simulink model "Model_ThreePhase_SixArm"  (R2022a)
settings: Solver=VariableStepAuto  StartTime=0.0  StopTime=10.0  RelTol=1e-3
libraries: fl_lib x45
settings Model: Creator=chack  LastModifiedBy=chack

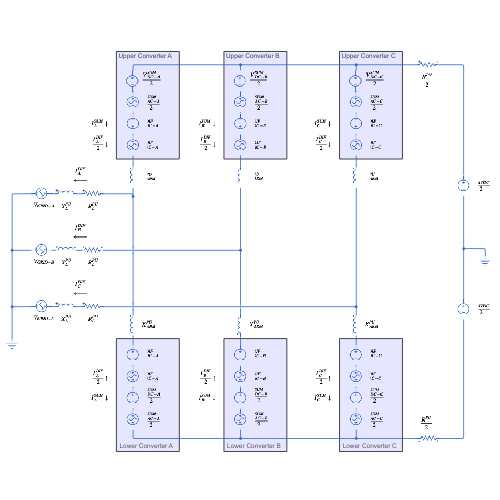
[thumbnail: Simulink's stored preview of the top-level diagram]
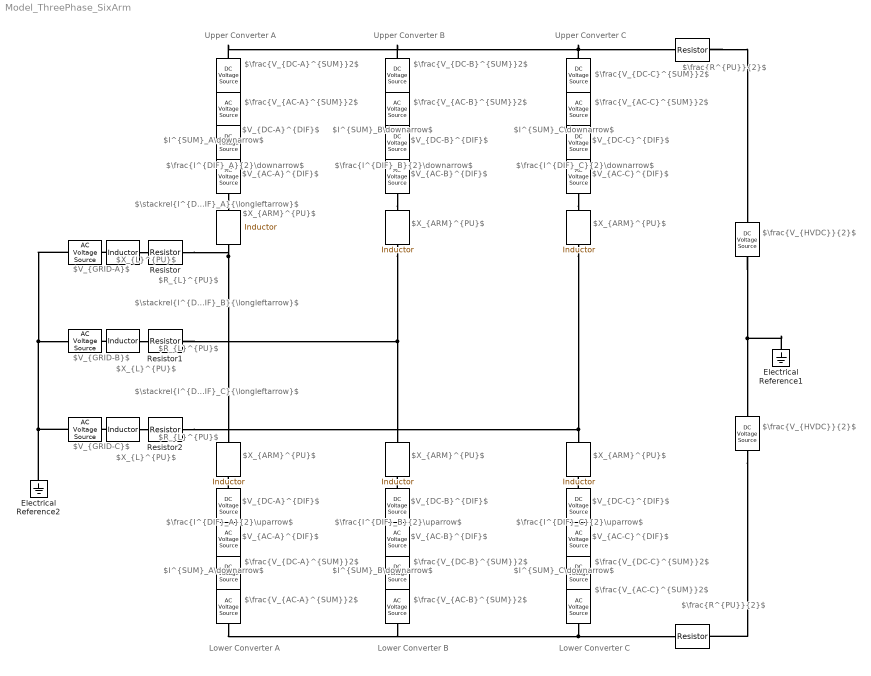
== system Model_ThreePhase_SixArm ==
  note: $I^{SUM}_A\downarrow$
  note: $\frac{I^{DIF}_A}{2}\downarrow$
  note: Lower Converter A
  note: Upper Converter A
  note: $V_{DC-A}^{DIF}$
  note: $\frac{V_{DC-A}^{SUM}}2$
  note: $V_{GRID-A}$
  note: $R_{L}^{PU}$
  note: $X_{L}^{PU}$
  note: $\frac{V_{HVDC}}{2}$
  note: $\frac{V_{HVDC}}{2}$
  note: $\frac{R^{PU}}{2}$
  note: $\frac{V_{AC-A}^{SUM}}2$
  note: $V_{AC-A}^{DIF}$
  note: $X_{ARM}^{PU}$
  note: $\frac{V_{DC-A}^{SUM}}2$
  note: $V_{DC-A}^{DIF}$
  note: $V_{AC-A}^{DIF}$
  note: $\frac{V_{AC-A}^{SUM}}2$
  note: $X_{ARM}^{PU}$
  note: $\frac{R^{PU}}{2}$
  note: $\stackrel{I^{DIF}_A}{\longleftarrow}$
  note: $\frac{I^{DIF}_A}{2}\uparrow$
  note: $I^{SUM}_A\downarrow$
  note: $X_{L}^{PU}$
  note: $V_{DC-B}^{DIF}$
  note: Lower Converter B
  note: $\frac{V_{AC-B}^{SUM}}2$
  note: $V_{AC-B}^{DIF}$
  note: $V_{DC-B}^{DIF}$
  note: $R_{L}^{PU}$
  note: $\frac{V_{AC-B}^{SUM}}2$
  note: $\frac{I^{DIF}_B}{2}\downarrow$
  note: $X_{ARM}^{PU}$
  note: $V_{AC-B}^{DIF}$
  note: $I^{SUM}_B\downarrow$
  note: $\frac{V_{DC-B}^{SUM}}2$
  note: $\frac{I^{DIF}_B}{2}\uparrow$
  note: Upper Converter B
  note: $\frac{V_{DC-B}^{SUM}}2$
  note: $X_{ARM}^{PU}$
  note: $\stackrel{I^{DIF}_B}{\longleftarrow}$
  note: $I^{SUM}_B\downarrow$
  note: $V_{GRID-B}$
  note: $X_{L}^{PU}$
  note: $V_{DC-C}^{DIF}$
  note: Lower Converter C
  note: $\frac{V_{AC-C}^{SUM}}2$
  note: $V_{AC-C}^{DIF}$
  note: $V_{DC-C}^{DIF}$
  note: $R_{L}^{PU}$
  note: $\frac{V_{AC-C}^{SUM}}2$
  note: $\frac{I^{DIF}_C}{2}\downarrow$
  note: $X_{ARM}^{PU}$
  note: $V_{AC-C}^{DIF}$
  note: $I^{SUM}_C\downarrow$
  note: $\frac{V_{DC-C}^{SUM}}2$
  note: $\frac{I^{DIF}_C}{2}\uparrow$
  note: Upper Converter C
  note: $\frac{V_{DC-C}^{SUM}}2$
  note: $X_{ARM}^{PU}$
  note: $\stackrel{I^{DIF}_C}{\longleftarrow}$
  note: $I^{SUM}_C\downarrow$
  note: $V_{GRID-C}$
  " " : fl_lib/Electrical/Electrical Sources/AC Voltage Source  amp=1 V  shift=0 deg  frequency=60 Hz  omega=0 rad/s
      settings: SourceProductBaseCode=PW,SS,VE
  "  " : fl_lib/Electrical/Electrical Elements/Inductor  l=1e-6 H  r=0 Ohm  g=1e-9 1/Ohm  i_specify=off  i_priority=None  i=0 A  i_nominal_specify=off  i_nominal_unit=A  i_nominal_value=1  v_specify=off  v_priority=None  v=0 V  v_nominal_specify=off  v_nominal_unit=V  v_nominal_value=1  i_L_specify=off  i_L_priority=High  i_L=0 A  i_L_nominal_specify=off  i_L_nominal_unit=A  i_L_nominal_value=1
      settings: SourceProductBaseCode=PW,SS,VE
  "   " : fl_lib/Electrical/Electrical Elements/Inductor  l=1e-6 H  r=0 Ohm  g=1e-9 1/Ohm  i_specify=off  i_priority=None  i=0 A  i_nominal_specify=off  i_nominal_unit=A  i_nominal_value=1  v_specify=off  v_priority=None  v=0 V  v_nominal_specify=off  v_nominal_unit=V  v_nominal_value=1  i_L_specify=off  i_L_priority=High  i_L=0 A  i_L_nominal_specify=off  i_L_nominal_unit=A  i_L_nominal_value=1
      settings: SourceProductBaseCode=PW,SS,VE
  "    " : fl_lib/Electrical/Electrical Sources/DC Voltage Source  v0=1 V
      settings: SourceProductBaseCode=PW,SS,VE
  "     " : fl_lib/Electrical/Electrical Sources/DC Voltage Source  v0=1 V
      settings: SourceProductBaseCode=PW,SS,VE
  "       " : fl_lib/Electrical/Electrical Elements/Resistor  R=1 Ohm  i_specify=off  i_priority=None  i=0 A  i_nominal_specify=off  i_nominal_unit=A  i_nominal_value=1  v_specify=off  v_priority=None  v=0 V  v_nominal_specify=off  v_nominal_unit=V  v_nominal_value=1
      settings: SourceProductBaseCode=PW,SS,VE
  "         " : fl_lib/Electrical/Electrical Elements/Resistor  R=1 Ohm  i_specify=off  i_priority=None  i=0 A  i_nominal_specify=off  i_nominal_unit=A  i_nominal_value=1  v_specify=off  v_priority=None  v=0 V  v_nominal_specify=off  v_nominal_unit=V  v_nominal_value=1
      settings: SourceProductBaseCode=PW,SS,VE
  "            " : fl_lib/Electrical/Electrical Sources/AC Voltage Source  amp=1 V  shift=0 deg  frequency=60 Hz  omega=0 rad/s
      settings: SourceProductBaseCode=PW,SS,VE
  "             " : fl_lib/Electrical/Electrical Sources/DC Voltage Source  v0=1 V
      settings: SourceProductBaseCode=PW,SS,VE
  "                " : fl_lib/Electrical/Electrical Sources/DC Voltage Source  v0=1 V
      settings: SourceProductBaseCode=PW,SS,VE
  "                 " : fl_lib/Electrical/Electrical Sources/AC Voltage Source  amp=1 V  shift=0 deg  frequency=60 Hz  omega=0 rad/s
      settings: SourceProductBaseCode=PW,SS,VE
  "                  " : fl_lib/Electrical/Electrical Sources/AC Voltage Source  amp=1 V  shift=0 deg  frequency=60 Hz  omega=0 rad/s
      settings: SourceProductBaseCode=PW,SS,VE
  "                   " : fl_lib/Electrical/Electrical Sources/AC Voltage Source  amp=1 V  shift=0 deg  frequency=60 Hz  omega=0 rad/s
      settings: SourceProductBaseCode=PW,SS,VE
  "                      " : fl_lib/Electrical/Electrical Elements/Inductor  l=1e-6 H  r=0 Ohm  g=1e-9 1/Ohm  i_specify=off  i_priority=None  i=0 A  i_nominal_specify=off  i_nominal_unit=A  i_nominal_value=1  v_specify=off  v_priority=None  v=0 V  v_nominal_specify=off  v_nominal_unit=V  v_nominal_value=1  i_L_specify=off  i_L_priority=High  i_L=0 A  i_L_nominal_specify=off  i_L_nominal_unit=A  i_L_nominal_value=1
      settings: SourceProductBaseCode=PW,SS,VE
  "                         " : fl_lib/Electrical/Electrical Sources/DC Voltage Source  v0=1 V
      settings: SourceProductBaseCode=PW,SS,VE
  "                             " : fl_lib/Electrical/Electrical Sources/DC Voltage Source  v0=1 V
      settings: SourceProductBaseCode=PW,SS,VE
  "                              " : fl_lib/Electrical/Electrical Sources/AC Voltage Source  amp=1 V  shift=0 deg  frequency=60 Hz  omega=0 rad/s
      settings: SourceProductBaseCode=PW,SS,VE
  "                                 " : fl_lib/Electrical/Electrical Sources/AC Voltage Source  amp=1 V  shift=0 deg  frequency=60 Hz  omega=0 rad/s
      settings: SourceProductBaseCode=PW,SS,VE
  "                                   " : fl_lib/Electrical/Electrical Elements/Inductor  l=1e-6 H  r=0 Ohm  g=1e-9 1/Ohm  i_specify=off  i_priority=None  i=0 A  i_nominal_specify=off  i_nominal_unit=A  i_nominal_value=1  v_specify=off  v_priority=None  v=0 V  v_nominal_specify=off  v_nominal_unit=V  v_nominal_value=1  i_L_specify=off  i_L_priority=High  i_L=0 A  i_L_nominal_specify=off  i_L_nominal_unit=A  i_L_nominal_value=1
      settings: SourceProductBaseCode=PW,SS,VE
  "                                    " : fl_lib/Electrical/Electrical Sources/DC Voltage Source  v0=1 V
      settings: SourceProductBaseCode=PW,SS,VE
  "                                     " : fl_lib/Electrical/Electrical Sources/AC Voltage Source  amp=1 V  shift=0 deg  frequency=60 Hz  omega=0 rad/s
      settings: SourceProductBaseCode=PW,SS,VE
  "                                        " : fl_lib/Electrical/Electrical Sources/DC Voltage Source  v0=1 V
      settings: SourceProductBaseCode=PW,SS,VE
  "                                         " : fl_lib/Electrical/Electrical Sources/AC Voltage Source  amp=1 V  shift=0 deg  frequency=60 Hz  omega=0 rad/s
      settings: SourceProductBaseCode=PW,SS,VE
  "                                           " : fl_lib/Electrical/Electrical Sources/AC Voltage Source  amp=1 V  shift=0 deg  frequency=60 Hz  omega=0 rad/s
      settings: SourceProductBaseCode=PW,SS,VE
  "                                              " : fl_lib/Electrical/Electrical Sources/DC Voltage Source  v0=1 V
      settings: SourceProductBaseCode=PW,SS,VE
  "                                                " : fl_lib/Electrical/Electrical Sources/AC Voltage Source  amp=1 V  shift=0 deg  frequency=60 Hz  omega=0 rad/s
      settings: SourceProductBaseCode=PW,SS,VE
  "                                                    " : fl_lib/Electrical/Electrical Elements/Inductor  l=1e-6 H  r=0 Ohm  g=1e-9 1/Ohm  i_specify=off  i_priority=None  i=0 A  i_nominal_specify=off  i_nominal_unit=A  i_nominal_value=1  v_specify=off  v_priority=None  v=0 V  v_nominal_specify=off  v_nominal_unit=V  v_nominal_value=1  i_L_specify=off  i_L_priority=High  i_L=0 A  i_L_nominal_specify=off  i_L_nominal_unit=A  i_L_nominal_value=1
      settings: SourceProductBaseCode=PW,SS,VE
  "                                                           " : fl_lib/Electrical/Electrical Sources/DC Voltage Source  v0=1 V
      settings: SourceProductBaseCode=PW,SS,VE
  "                                                            " : fl_lib/Electrical/Electrical Sources/AC Voltage Source  amp=1 V  shift=0 deg  frequency=60 Hz  omega=0 rad/s
      settings: SourceProductBaseCode=PW,SS,VE
  "                                                             " : fl_lib/Electrical/Electrical Sources/DC Voltage Source  v0=1 V
      settings: SourceProductBaseCode=PW,SS,VE
  "                                                                 " : fl_lib/Electrical/Electrical Sources/AC Voltage Source  amp=1 V  shift=0 deg  frequency=60 Hz  omega=0 rad/s
      settings: SourceProductBaseCode=PW,SS,VE
  "                                                                      " : fl_lib/Electrical/Electrical Sources/AC Voltage Source  amp=1 V  shift=0 deg  frequency=60 Hz  omega=0 rad/s
      settings: SourceProductBaseCode=PW,SS,VE
  "                                                                         " : fl_lib/Electrical/Electrical Elements/Inductor  l=1e-6 H  r=0 Ohm  g=1e-9 1/Ohm  i_specify=off  i_priority=None  i=0 A  i_nominal_specify=off  i_nominal_unit=A  i_nominal_value=1  v_specify=off  v_priority=None  v=0 V  v_nominal_specify=off  v_nominal_unit=V  v_nominal_value=1  i_L_specify=off  i_L_priority=High  i_L=0 A  i_L_nominal_specify=off  i_L_nominal_unit=A  i_L_nominal_value=1
      settings: SourceProductBaseCode=PW,SS,VE
  "                                                                           " : fl_lib/Electrical/Electrical Sources/AC Voltage Source  amp=1 V  shift=0 deg  frequency=60 Hz  omega=0 rad/s
      settings: SourceProductBaseCode=PW,SS,VE
  "                                                                            " : fl_lib/Electrical/Electrical Sources/DC Voltage Source  v0=1 V
      settings: SourceProductBaseCode=PW,SS,VE
  "                                                                             " : fl_lib/Electrical/Electrical Elements/Inductor  l=1e-6 H  r=0 Ohm  g=1e-9 1/Ohm  i_specify=off  i_priority=None  i=0 A  i_nominal_specify=off  i_nominal_unit=A  i_nominal_value=1  v_specify=off  v_priority=None  v=0 V  v_nominal_specify=off  v_nominal_unit=V  v_nominal_value=1  i_L_specify=off  i_L_priority=High  i_L=0 A  i_L_nominal_specify=off  i_L_nominal_unit=A  i_L_nominal_value=1
      settings: SourceProductBaseCode=PW,SS,VE
  "                                                                                                    " : fl_lib/Electrical/Electrical Sources/DC Voltage Source  v0=1 V
      settings: SourceProductBaseCode=PW,SS,VE
  "                                                                                                                  " : fl_lib/Electrical/Electrical Sources/DC Voltage Source  v0=1 V
      settings: SourceProductBaseCode=PW,SS,VE
  "                                                                                                                    " : fl_lib/Electrical/Electrical Elements/Inductor  l=1e-6 H  r=0 Ohm  g=1e-9 1/Ohm  i_specify=off  i_priority=None  i=0 A  i_nominal_specify=off  i_nominal_unit=A  i_nominal_value=1  v_specify=off  v_priority=None  v=0 V  v_nominal_specify=off  v_nominal_unit=V  v_nominal_value=1  i_L_specify=off  i_L_priority=High  i_L=0 A  i_L_nominal_specify=off  i_L_nominal_unit=A  i_L_nominal_value=1
      settings: SourceProductBaseCode=PW,SS,VE
  "                                                                                                                                    " : fl_lib/Electrical/Electrical Elements/Inductor  l=1e-6 H  r=0 Ohm  g=1e-9 1/Ohm  i_specify=off  i_priority=None  i=0 A  i_nominal_specify=off  i_nominal_unit=A  i_nominal_value=1  v_specify=off  v_priority=None  v=0 V  v_nominal_specify=off  v_nominal_unit=V  v_nominal_value=1  i_L_specify=off  i_L_priority=High  i_L=0 A  i_L_nominal_specify=off  i_L_nominal_unit=A  i_L_nominal_value=1
      settings: SourceProductBaseCode=PW,SS,VE
  Electrical Reference1 : fl_lib/Electrical/Electrical Elements/Electrical Reference
      settings: SourceProductBaseCode=PW,SS,VE
  Electrical Reference2 : fl_lib/Electrical/Electrical Elements/Electrical Reference
      settings: SourceProductBaseCode=PW,SS,VE
  Resistor : fl_lib/Electrical/Electrical Elements/Resistor  R=1 Ohm  i_specify=off  i_priority=None  i=0 A  i_nominal_specify=off  i_nominal_unit=A  i_nominal_value=1  v_specify=off  v_priority=None  v=0 V  v_nominal_specify=off  v_nominal_unit=V  v_nominal_value=1
      settings: SourceProductBaseCode=PW,SS,VE
  Resistor1 : fl_lib/Electrical/Electrical Elements/Resistor  R=1 Ohm  i_specify=off  i_priority=None  i=0 A  i_nominal_specify=off  i_nominal_unit=A  i_nominal_value=1  v_specify=off  v_priority=None  v=0 V  v_nominal_specify=off  v_nominal_unit=V  v_nominal_value=1
      settings: SourceProductBaseCode=PW,SS,VE
  Resistor2 : fl_lib/Electrical/Electrical Elements/Resistor  R=1 Ohm  i_specify=off  i_priority=None  i=0 A  i_nominal_specify=off  i_nominal_unit=A  i_nominal_value=1  v_specify=off  v_priority=None  v=0 V  v_nominal_specify=off  v_nominal_unit=V  v_nominal_value=1
      settings: SourceProductBaseCode=PW,SS,VE
  connections:
  "            "/LConn1 -- "                "/RConn1
  "     "/RConn1 -- Electrical Reference1/LConn1 -- "    "/LConn1
  "       "/RConn1 -- "     "/LConn1
  "  "/LConn1 -- " "/LConn1
  "  "/RConn1 -- Resistor/LConn1
  "             "/RConn1 -- "            "/RConn1
  "                 "/RConn1 -- "             "/LConn1
  Resistor/RConn1 -- "   "/LConn1 -- "                                                    "/RConn1
  "                  "/LConn1 -- "                             "/RConn1
  "                                 "/LConn1 -- "                         "/RConn1
  "                         "/LConn1 -- "                                                    "/LConn1
  "                             "/LConn1 -- "                                 "/RConn1
  "    "/RConn1 -- "         "/LConn1
  "                 "/LConn1 -- "   "/RConn1
  "                      "/LConn1 -- Resistor1/RConn1 -- "                                                                         "/RConn1
  "                                    "/LConn1 -- "                                                            "/RConn1
  "                                   "/LConn1 -- "                                         "/LConn1
  "                                           "/RConn1 -- "                                        "/LConn1
  "                                                            "/LConn1 -- "                                                                                                    "/RConn1
  "                                           "/LConn1 -- "                      "/RConn1
  "                              "/LConn1 -- "                                    "/RConn1
  "                                        "/RConn1 -- "                                     "/RConn1
  Electrical Reference2/LConn1 -- "                   "/RConn1 -- " "/RConn1 -- "                                         "/RConn1
  "                                     "/LConn1 -- "                                              "/RConn1
  "                                   "/RConn1 -- Resistor1/LConn1
  "                                                                                                    "/LConn1 -- "                                                                         "/LConn1
  "                                                                                                                                    "/RConn1 -- "                                                                                                                    "/LConn1 -- Resistor2/RConn1
  "                                                             "/LConn1 -- "                                                "/RConn1
  "                                                                             "/LConn1 -- "                   "/LConn1
  "                                                                      "/RConn1 -- "                                                           "/LConn1
  "                                                "/LConn1 -- "                                                                                                                  "/RConn1
  "                                                                      "/LConn1 -- "                                                                                                                    "/RConn1
  "                                                                           "/LConn1 -- "                                                             "/RConn1
  "                                                           "/RConn1 -- "                                                                 "/RConn1
  "                                                                 "/LConn1 -- "                                                                            "/RConn1
  "                                                                             "/RConn1 -- Resistor2/LConn1
  "                                                                                                                  "/LConn1 -- "                                                                                                                                    "/LConn1
  "                                                                            "/LConn1 -- "                "/LConn1 -- "                                              "/LConn1 -- "       "/LConn1
  "                                                                           "/RConn1 -- "                  "/RConn1 -- "                              "/RConn1 -- "         "/RConn1
